simulink library "aerosimlib"  (Simulink 5.0)
values from neighbouring files (symbols this model uses):
  stdatm = [0 100 200 300 400 500 600 700 800 900 1000 1100 ... (4305 elements, 861x5)]    [stdatm.mat]
undefined symbols (not defined in the file or in its folder): AlphaBnd, b, BetaBnd, CDda, CDde, CDdf, CDdr, CDM, CDmin, CGempty, CGgross, CL0, CLa, CLalphadot, Clbeta, Clda, CLde, CLdf, Cldr, CLM, CLmind, Clp, CLq, Clr, Cm0, Cma, Cmalphadot, Cmde, Cmdf, CmM, Cmq, Cnbeta, Cnda, Cndr, Cnp, Cnr, CP, CT, CYbeta, CYda, CYdr, CYp, CYr, Displacement, dmy, Engine, EulerIni, FuelFlow, FuelIni, J, Jempty, Jeng, Jgross, Jprop, MAC, MAP, MAPLim, MassIni, MaxPower, mempty ... (+25)
libraries: aerosimlib x350, simulink3 x41
(part 5 of 10)

== system aerosimlib/Sensors/Noise Correlation ==
  Gauss-Markov  Process : Subsystem  mask(Gauss-Markov Process){beta=, seed=, Var=, T=}
      mask prompts: beta "Time constant:"; seed "White-noise seed:"; Var "Variance:"; T "Sample time:"
      mask help: The Gauss-Markov process has an exponentially decreasing autocorrelation function.
      mask Help:
      | <P>The Gauss-Markov process has an exponentially decreasing autocorrelation function.</P>
      | <P><B>Block parameters:</B>
      | <LI>Time constant = the noise correlation time.
      | <LI>White-noise seed = the starting seed of the white-noise source.
      | <LI>Variance = the variance of the white-noise source.
      | <LI>Sample time = the sample time of the white-noise source.
      | </P>
  Random Walk : Subsystem  mask(Random Walk){seed=, Var=, T=}
      mask prompts: seed "White-noise seed:"; Var "Variance:"; T "Sample time:"
      mask help: The random walk is also known as the Wiener process or Brownian motion. Essentially, this is the integral of a random noise signal.
      mask Help:
      | <P>The random walk is also known as the Wiener process or Brownian motion. Essentially, this is the integral of a random noise signal.</P>
      | <P><B>Block parameters:</B>
      | <LI>White-noise seed = the starting seed of the white-noise source.
      | <LI>Variance = the variance of the white-noise source.
      | <LI>Sample time = the sample time of the white-noise source.
      | </P>

== system aerosimlib/Transformations/Body-Inertial DCM From Euler Angles ==
  note: Sources
  note: Assemble Body-Inertial DCM
  note: Output
  note: Attitude trigonometry
  Euler : Inport  PortDimensions=[3 1]
  -sin(theta) : Gain  Gain=-1  SaturateOnIntegerOverflow=on
  Demux : Demux  Outputs=3
  Math Function : Math  Operator=transpose
  Rbi Matrix : simulink3/Signals & Systems/Matrix Concatenation  numInports=3  catMethod=Horizontal
  Rbi Col1 : simulink3/Signals & Systems/Matrix Concatenation  numInports=3  catMethod=Vertical
  Rbi Col2 : simulink3/Signals & Systems/Matrix Concatenation  numInports=3  catMethod=Vertical
  Rbi Col3 : simulink3/Signals & Systems/Matrix Concatenation  numInports=3  catMethod=Vertical
  Sum2 : Sum  Inputs=+-  SaturateOnIntegerOverflow=on  InputSameDT=on
  Sum3 : Sum  SaturateOnIntegerOverflow=on  InputSameDT=on
  Sum4 : Sum  SaturateOnIntegerOverflow=on  InputSameDT=on
  Sum5 : Sum  Inputs=+-  SaturateOnIntegerOverflow=on  InputSameDT=on
  cos(phi) : Trigonometry  Operator=cos
  cos(phi)cos(psi) : Product  SaturateOnIntegerOverflow=on  InputSameDT=on
  cos(phi)cos(theta) : Product  SaturateOnIntegerOverflow=on  InputSameDT=on
  cos(phi)sin(psi) : Product  SaturateOnIntegerOverflow=on  InputSameDT=on
  cos(phi)sin(theta)cos(psi) : Product  Inputs=3  SaturateOnIntegerOverflow=on  InputSameDT=on
  cos(phi)sin(theta)sin(psi) : Product  Inputs=3  SaturateOnIntegerOverflow=on  InputSameDT=on
  cos(psi) : Trigonometry  Operator=cos
  cos(theta) : Trigonometry  Operator=cos
  cos(theta)cos(psi) : Product  SaturateOnIntegerOverflow=on  InputSameDT=on
  cos(theta)sin(psi) : Product  SaturateOnIntegerOverflow=on  InputSameDT=on
  sin(phi) : Trigonometry
  sin(phi)cos(psi) : Product  SaturateOnIntegerOverflow=on  InputSameDT=on
  sin(phi)cos(theta) : Product  SaturateOnIntegerOverflow=on  InputSameDT=on
  sin(phi)sin(psi) : Product  SaturateOnIntegerOverflow=on  InputSameDT=on
  sin(phi)sin(theta)cos(psi) : Product  Inputs=3  SaturateOnIntegerOverflow=on  InputSameDT=on
  sin(phi)sin(theta)sin(psi) : Product  Inputs=3  SaturateOnIntegerOverflow=on  InputSameDT=on
  sin(psi) : Trigonometry
  sin(theta) : Trigonometry
  DCM : Outport
  wires:
  Euler/1 -> Demux/1
  Rbi Col1/1 -> Rbi Matrix/1
  Rbi Col2/1 -> Rbi Matrix/2
  Rbi Col3/1 -> Rbi Matrix/3
  Rbi Matrix/1 -> Math Function/1
  Demux/1 -> sin(phi)/1, cos(phi)/1
  Demux/2 -> cos(theta)/1, sin(theta)/1
  Demux/3 -> cos(psi)/1, sin(psi)/1
  sin(phi)/1 -> sin(phi)sin(psi)/1, sin(phi)cos(psi)/1, sin(phi)sin(theta)sin(psi)/1, sin(phi)cos(theta)/1, sin(phi)sin(theta)cos(psi)/1
  cos(phi)/1 -> cos(phi)cos(theta)/1, cos(phi)sin(theta)sin(psi)/1, cos(phi)sin(theta)cos(psi)/1, cos(phi)cos(psi)/1, cos(phi)sin(psi)/1
  sin(theta)/1 -> cos(phi)sin(theta)cos(psi)/2, cos(phi)sin(theta)sin(psi)/2, sin(phi)sin(theta)sin(psi)/2, sin(phi)sin(theta)cos(psi)/2, -sin(theta)/1
  cos(theta)/1 -> cos(phi)cos(theta)/2, sin(phi)cos(theta)/2, cos(theta)sin(psi)/1, cos(theta)cos(psi)/1
  sin(psi)/1 -> sin(phi)sin(psi)/2, cos(phi)sin(theta)sin(psi)/3, sin(phi)sin(theta)sin(psi)/3, cos(phi)sin(psi)/2, cos(theta)sin(psi)/2
  cos(psi)/1 -> sin(phi)cos(psi)/2, cos(phi)sin(theta)cos(psi)/3, cos(phi)cos(psi)/2, sin(phi)sin(theta)cos(psi)/3, cos(theta)cos(psi)/2
  cos(phi)sin(psi)/1 -> Sum2/2
  cos(phi)cos(psi)/1 -> Sum3/2
  sin(phi)sin(theta)cos(psi)/1 -> Sum2/1
  cos(phi)sin(theta)cos(psi)/1 -> Sum4/1
  sin(phi)sin(psi)/1 -> Sum4/2
  cos(phi)sin(theta)sin(psi)/1 -> Sum5/1
  sin(phi)cos(psi)/1 -> Sum5/2
  cos(theta)cos(psi)/1 -> Rbi Col1/1
  cos(theta)sin(psi)/1 -> Rbi Col1/2
  -sin(theta)/1 -> Rbi Col1/3
  Sum2/1 -> Rbi Col2/1
  Sum3/1 -> Rbi Col2/2
  sin(phi)cos(theta)/1 -> Rbi Col2/3
  Sum4/1 -> Rbi Col3/1
  Sum5/1 -> Rbi Col3/2
  cos(phi)cos(theta)/1 -> Rbi Col3/3
  Math Function/1 -> DCM/1
  sin(phi)sin(theta)sin(psi)/1 -> Sum3/1

== system aerosimlib/Transformations/Body-Inertial DCM From Quaternions ==
  note: Output
  note: Quaternion products
  note: Assemble Body-Inertial DCM
  note: Sources
  Quaternions : Inport  PortDimensions=[4 1]
  Demux : Demux
  Demux1 : Demux
  Gain{,1..5} (6 alike) : Gain  Gain=2  SaturateOnIntegerOverflow=on
  Get DCM : Math  Operator=transpose
  Math Function : Math  Operator=square
  Rbi Matrix : simulink3/Signals & Systems/Matrix Concatenation  numInports=3  catMethod=Horizontal
  Rbi Col1 : simulink3/Signals & Systems/Matrix Concatenation  numInports=3  catMethod=Vertical
  Rbi Col2 : simulink3/Signals & Systems/Matrix Concatenation  numInports=3  catMethod=Vertical
  Rbi Col3 : simulink3/Signals & Systems/Matrix Concatenation  numInports=3  catMethod=Vertical
  Sum : Sum  Inputs=++--  SaturateOnIntegerOverflow=on  InputSameDT=on
  Sum1 : Sum  SaturateOnIntegerOverflow=on  InputSameDT=on
  Sum2 : Sum  Inputs=+-  SaturateOnIntegerOverflow=on  InputSameDT=on
  Sum3 : Sum  Inputs=+-  SaturateOnIntegerOverflow=on  InputSameDT=on
  Sum4 : Sum  Inputs=+-+-  SaturateOnIntegerOverflow=on  InputSameDT=on
  Sum5 : Sum  SaturateOnIntegerOverflow=on  InputSameDT=on
  Sum6 : Sum  SaturateOnIntegerOverflow=on  InputSameDT=on
  Sum7 : Sum  Inputs=+-  SaturateOnIntegerOverflow=on  InputSameDT=on
  Sum8 : Sum  Inputs=+--+  SaturateOnIntegerOverflow=on  InputSameDT=on
  exe0 : Product  SaturateOnIntegerOverflow=on  InputSameDT=on
  exey : Product  SaturateOnIntegerOverflow=on  InputSameDT=on
  exez : Product  SaturateOnIntegerOverflow=on  InputSameDT=on
  eye0 : Product  SaturateOnIntegerOverflow=on  InputSameDT=on
  eyez : Product  SaturateOnIntegerOverflow=on  InputSameDT=on
  eze0 : Product  SaturateOnIntegerOverflow=on  InputSameDT=on
  DCM : Outport
  wires:
  Get DCM/1 -> DCM/1
  Rbi Matrix/1 -> Get DCM/1
  Sum8/1 -> Rbi Col3/3
  Gain5/1 -> Rbi Col3/2
  Gain4/1 -> Rbi Col3/1
  Rbi Col3/1 -> Rbi Matrix/3
  Sum7/1 -> Gain5/1
  Sum6/1 -> Gain4/1
  Rbi Col2/1 -> Rbi Matrix/2
  Gain3/1 -> Rbi Col2/3
  Sum4/1 -> Rbi Col2/2
  Gain2/1 -> Rbi Col2/1
  Sum5/1 -> Gain3/1
  Sum3/1 -> Gain2/1
  Rbi Col1/1 -> Rbi Matrix/1
  Gain1/1 -> Rbi Col1/3
  Gain/1 -> Rbi Col1/2
  Sum/1 -> Rbi Col1/1
  Sum2/1 -> Gain1/1
  Sum1/1 -> Gain/1
  exe0/1 -> Sum5/2, Sum7/2
  eyez/1 -> Sum5/1, Sum7/1
  eye0/1 -> Sum2/2, Sum6/2
  exez/1 -> Sum2/1, Sum6/1
  eze0/1 -> Sum1/2, Sum3/2
  exey/1 -> Sum1/1, Sum3/1
  Math Function/1 -> Demux1/1
  Demux/4 -> eze0/1, exez/2, eyez/2
  Demux/3 -> exey/2, eye0/1, eyez/1
  Demux/2 -> exey/1, exez/1, exe0/1
  Demux/1 -> eze0/2, eye0/2, exe0/2
  Quaternions/1 -> Math Function/1, Demux/1
  Demux1/1 -> Sum/1, Sum4/1, Sum8/1
  Demux1/2 -> Sum/2, Sum4/2, Sum8/2
  Demux1/3 -> Sum/3, Sum4/3, Sum8/3
  Demux1/4 -> Sum/4, Sum4/4, Sum8/4

== system aerosimlib/Transformations/Body-Wind DCM ==
  note: Output
  note: Assemble Body-Wind DCM
  note: Trigonometric functions
  note: Sources
  WindAxesVel : Inport  PortDimensions=[3 1]
  ChSign : Gain  Gain=-1  SaturateOnIntegerOverflow=on
  ChSign1 : Gain  Gain=-1  SaturateOnIntegerOverflow=on
  ChSign2 : Gain  Gain=-1  SaturateOnIntegerOverflow=on
  Demux : Demux  Outputs=3
  Product{,1..3} (4 alike) : Product  SaturateOnIntegerOverflow=on  InputSameDT=on
  S Matrix : simulink3/Signals & Systems/Matrix Concatenation  numInports=3  catMethod=Horizontal
  S Col1 : simulink3/Signals & Systems/Matrix Concatenation  numInports=3  catMethod=Vertical
  S Col2 : simulink3/Signals & Systems/Matrix Concatenation  numInports=3  catMethod=Vertical
  S Col3 : simulink3/Signals & Systems/Matrix Concatenation  numInports=3  catMethod=Vertical
  Terminator : Terminator
  Trigonometric Function : Trigonometry
  Trigonometric Function1 : Trigonometry  Operator=cos
  Trigonometric Function2 : Trigonometry
  Trigonometric Function3 : Trigonometry  Operator=cos
  Zero : Constant  Value=0
  DCM : Outport
  wires:
  S Matrix/1 -> DCM/1
  S Col3/1 -> S Matrix/3
  S Col2/1 -> S Matrix/2
  S Col1/1 -> S Matrix/1
  ChSign2/1 -> S Col3/2
  Product2/1 -> S Col3/1
  Product3/1 -> ChSign2/1
  Zero/1 -> S Col2/3
  ChSign1/1 -> S Col1/3
  ChSign/1 -> S Col1/2
  Product/1 -> S Col1/1
  Product1/1 -> ChSign/1
  Trigonometric Function3/1 -> Product/2, S Col2/2, Product2/2
  Trigonometric Function2/1 -> Product1/2, S Col2/1, Product3/2
  Trigonometric Function1/1 -> Product/1, Product1/1, S Col3/3
  Trigonometric Function/1 -> ChSign1/1, Product2/1, Product3/1
  Demux/1 -> Terminator/1
  WindAxesVel/1 -> Demux/1
  Demux/2 -> Trigonometric Function3/1, Trigonometric Function2/1
  Demux/3 -> Trigonometric Function/1, Trigonometric Function1/1

== system aerosimlib/Transformations/Body2LTP ==
  VecB : Inport
  Euler : Inport  Port=2
  Fcn : Fcn  Expr=cos(u(5))*u(1) + sin(u(4))*sin(u(5))*u(2) + cos(u(4))*sin(u(5))*u(3)
  Fcn1 : Fcn  Expr=cos(u(4))*u(2) - sin(u(4))*u(3)
  Fcn2 : Fcn  Expr=-sin(u(5))*u(1) + sin(u(4))*cos(u(5))*u(2) + cos(u(4))*cos(u(5))*u(3)
  Mux : Mux  Inputs=2
  Mux1 : Mux  Inputs=3
  VecLTP : Outport
  wires:
  Mux1/1 -> VecLTP/1
  Fcn2/1 -> Mux1/3
  Fcn1/1 -> Mux1/2
  Fcn/1 -> Mux1/1
  Mux/1 -> Fcn1/1, Fcn2/1, Fcn/1
  Euler/1 -> Mux/2
  VecB/1 -> Mux/1

== system aerosimlib/Transformations/ECEF Position ==
  note: Trigonometric functions
  note: Sources
  note: Output
  LLA : Inport  PortDimensions=[3 1]
  Demux : Demux  Outputs=3
  Equatorial Radius : Constant  Value=6378137
  First Eccentricity : Constant  Value=0.0818191908426
  Mux : Mux  Inputs=3
  One : Constant
  Product : Product  Inputs=3  SaturateOnIntegerOverflow=on  InputSameDT=on
  Product1 : Product  Inputs=3  SaturateOnIntegerOverflow=on  InputSameDT=on
  Product3 : Product  SaturateOnIntegerOverflow=on  InputSameDT=on
  Product4 : Product  SaturateOnIntegerOverflow=on  InputSameDT=on
  Product5 : Product  Inputs=*/  SaturateOnIntegerOverflow=on  InputSameDT=on
  Product6 : Product  SaturateOnIntegerOverflow=on  InputSameDT=on
  Sum : Sum  Inputs=|++  SaturateOnIntegerOverflow=on  InputSameDT=on
  Sum1 : Sum  Inputs=++|  SaturateOnIntegerOverflow=on  InputSameDT=on
  Sum2 : Sum  Inputs=|+-  SaturateOnIntegerOverflow=on  InputSameDT=on
  Sum3 : Sum  Inputs=|+-  SaturateOnIntegerOverflow=on  InputSameDT=on
  Trigonometric Function : Trigonometry
  Trigonometric Function1 : Trigonometry  Operator=cos
  Trigonometric Function2 : Trigonometry
  Trigonometric Function3 : Trigonometry  Operator=cos
  eps^2 : Math  Operator=square
  sin(phi)^2 : Math  Operator=square
  sqrt : Math  Operator=sqrt
  ECEF : Outport
  wires:
  Mux/1 -> ECEF/1
  Product1/1 -> Mux/2
  Product/1 -> Mux/1
  Trigonometric Function3/1 -> Product/3
  Trigonometric Function2/1 -> Product1/3
  Trigonometric Function1/1 -> Product/2, Product1/2
  LLA/1 -> Demux/1
  Demux/1 -> Trigonometric Function1/1, Trigonometric Function/1
  Demux/2 -> Trigonometric Function2/1, Trigonometric Function3/1
  Product5/1 -> Product4/1, Sum1/2
  sqrt/1 -> Product5/2
  Equatorial Radius/1 -> Product5/1
  Sum3/1 -> sqrt/1
  Product6/1 -> Sum3/2
  sin(phi)^2/1 -> Product6/1
  Product4/1 -> Sum/2
  First Eccentricity/1 -> eps^2/1
  One/1 -> Sum3/1, Sum2/1
  eps^2/1 -> Product6/2, Sum2/2
  Sum2/1 -> Product4/2
  Sum/1 -> Product3/1
  Product3/1 -> Mux/3
  Demux/3 -> Sum1/1, Sum/1
  Sum1/1 -> Product/1, Product1/1
  Trigonometric Function/1 -> sin(phi)^2/1, Product3/2

== system aerosimlib/Transformations/Euler Angles From Quaternions ==
  note: Compute Euler angles
  note: Sources
  note: Quaternion products
  Quaternions : Inport  PortDimensions=[4 1]
  2pi Bound : aerosimlib/Math/2pi Bound
  Demux : Demux
  Demux1 : Demux
  Gain6 : Gain  Gain=2  SaturateOnIntegerOverflow=on
  Gain7 : Gain  Gain=2  SaturateOnIntegerOverflow=on
  Gain8 : Gain  Gain=2  SaturateOnIntegerOverflow=on
  Math Function : Math  Operator=square
  Mux : Mux  Inputs=3
  Sum10 : Sum  Inputs=+--+  SaturateOnIntegerOverflow=on  InputSameDT=on
  Sum11 : Sum  Inputs=-+  SaturateOnIntegerOverflow=on  InputSameDT=on
  Sum12 : Sum  SaturateOnIntegerOverflow=on  InputSameDT=on
  Sum13 : Sum  Inputs=++--  SaturateOnIntegerOverflow=on  InputSameDT=on
  Sum9 : Sum  SaturateOnIntegerOverflow=on  InputSameDT=on
  Trigonometric Function : Trigonometry  Operator=atan2
  Trigonometric Function1 : Trigonometry  Operator=asin
  Trigonometric Function2 : Trigonometry  Operator=atan2
  exe0 : Product  SaturateOnIntegerOverflow=on  InputSameDT=on
  exey : Product  SaturateOnIntegerOverflow=on  InputSameDT=on
  exez : Product  SaturateOnIntegerOverflow=on  InputSameDT=on
  eye0 : Product  SaturateOnIntegerOverflow=on  InputSameDT=on
  eyez : Product  SaturateOnIntegerOverflow=on  InputSameDT=on
  eze0 : Product  SaturateOnIntegerOverflow=on  InputSameDT=on
  pi Bound : aerosimlib/Math/pi Bound
  pi Bound1 : aerosimlib/Math/pi Bound
  Euler : Outport
  wires:
  Sum9/1 -> Gain6/1
  Gain6/1 -> Trigonometric Function/1
  Sum10/1 -> Trigonometric Function/2
  Sum11/1 -> Gain7/1
  Gain7/1 -> Trigonometric Function1/1
  Sum12/1 -> Gain8/1
  Gain8/1 -> Trigonometric Function2/1
  Sum13/1 -> Trigonometric Function2/2
  Trigonometric Function1/1 -> pi Bound1/1
  Trigonometric Function/1 -> pi Bound/1
  Trigonometric Function2/1 -> 2pi Bound/1
  Quaternions/1 -> Math Function/1, Demux/1
  Demux/1 -> eze0/2, eye0/2, exe0/2
  Demux/2 -> exey/1, exez/1, exe0/1
  Demux/3 -> exey/2, eye0/1, eyez/1
  Demux/4 -> eze0/1, exez/2, eyez/2
  Demux1/1 -> Sum10/1, Sum13/1
  Demux1/2 -> Sum10/2, Sum13/2
  Demux1/3 -> Sum10/3, Sum13/3
  Demux1/4 -> Sum10/4, Sum13/4
  Math Function/1 -> Demux1/1
  exey/1 -> Sum12/1
  eze0/1 -> Sum12/2
  exez/1 -> Sum11/1
  eye0/1 -> Sum11/2
  eyez/1 -> Sum9/1
  exe0/1 -> Sum9/2
  Mux/1 -> Euler/1
  pi Bound/1 -> Mux/1
  pi Bound1/1 -> Mux/2
  2pi Bound/1 -> Mux/3

== system aerosimlib/Transformations/Euler Angles  From DCM ==
  DCM : Inport  PortDimensions=[3 3]
  C12 : Selector  InputType=Matrix  Elements=[1 3]  Columns=2  InputPortWidth=3
  C13 : Selector  InputType=Matrix  Elements=[1 3]  Columns=3  InputPortWidth=3
  C23 : Selector  InputType=Matrix  Elements=[1 3]  Rows=2  Columns=3  InputPortWidth=3
  ChSign : Gain  Gain=-1  SaturateOnIntegerOverflow=on
  Mux3 : Mux  Inputs=3
  Product2 : Product  Inputs=*/  SaturateOnIntegerOverflow=on  InputSameDT=on
  Product3 : Product  Inputs=*/  SaturateOnIntegerOverflow=on  InputSameDT=on
  Trigonometric Function : Trigonometry  Operator=asin
  Trigonometric Function1 : Trigonometry  Operator=cos
  Trigonometric Function2 : Trigonometry  Operator=asin
  Trigonometric Function3 : Trigonometry  Operator=asin
  Euler : Outport
  wires:
  DCM/1 -> C12/1, C23/1, C13/1
  Mux3/1 -> Euler/1
  Trigonometric Function3/1 -> Mux3/1
  Trigonometric Function2/1 -> Mux3/3
  Product2/1 -> Trigonometric Function2/1
  Product3/1 -> Trigonometric Function3/1
  C23/1 -> Product3/1
  Trigonometric Function1/1 -> Product3/2, Product2/2
  C12/1 -> Product2/1
  Trigonometric Function/1 -> Mux3/2, Trigonometric Function1/1
  ChSign/1 -> Trigonometric Function/1
  C13/1 -> ChSign/1

== system aerosimlib/Transformations/LTP2Body ==
  VecLTP : Inport
  Euler : Inport  Port=2
  Fcn : Fcn  Expr=cos(u(5))*u(1) - sin(u(5))*u(3)
  Fcn1 : Fcn  Expr=sin(u(4))*sin(u(5))*u(1) + cos(u(4))*u(2) + sin(u(4))*cos(u(5))*u(3)
  Fcn2 : Fcn  Expr=cos(u(4))*sin(u(5))*u(1) - sin(u(4))*u(2) + cos(u(4))*cos(u(5))*u(3)
  Mux : Mux  Inputs=2
  Mux1 : Mux  Inputs=3
  VecB : Outport
  wires:
  Mux1/1 -> VecB/1
  Fcn2/1 -> Mux1/3
  Fcn1/1 -> Mux1/2
  Fcn/1 -> Mux1/1
  Mux/1 -> Fcn1/1, Fcn2/1, Fcn/1
  Euler/1 -> Mux/2
  VecLTP/1 -> Mux/1

== system aerosimlib/Transformations/Quaternions From Euler Angles ==
  note: Sources
  note: Attitude trigonometry
  note: Compute quaternions
  note: Outputs
  Euler : Inport  PortDimensions=[3 1]
  1/2 : Gain  Gain=1/2  SaturateOnIntegerOverflow=on
  CCC : Product  Inputs=3  SaturateOnIntegerOverflow=on  InputSameDT=on
  CCS : Product  Inputs=3  SaturateOnIntegerOverflow=on  InputSameDT=on
  CSC : Product  Inputs=3  SaturateOnIntegerOverflow=on  InputSameDT=on
  CSS : Product  Inputs=3  SaturateOnIntegerOverflow=on  InputSameDT=on
  Demux : Demux  Outputs=3
  Mux : Mux
  SCC : Product  Inputs=3  SaturateOnIntegerOverflow=on  InputSameDT=on
  SCS : Product  Inputs=3  SaturateOnIntegerOverflow=on  InputSameDT=on
  SSC : Product  Inputs=3  SaturateOnIntegerOverflow=on  InputSameDT=on
  SSS : Product  Inputs=3  SaturateOnIntegerOverflow=on  InputSameDT=on
  Sum1 : Sum  SaturateOnIntegerOverflow=on  InputSameDT=on
  Sum2 : Sum  Inputs=+-  SaturateOnIntegerOverflow=on  InputSameDT=on
  Sum3 : Sum  Inputs=+-  SaturateOnIntegerOverflow=on  InputSameDT=on
  Sum9 : Sum  SaturateOnIntegerOverflow=on  InputSameDT=on
  cos(phi/2) : Trigonometry  Operator=cos
  cos(psi/2) : Trigonometry  Operator=cos
  cos(theta/2) : Trigonometry  Operator=cos
  sin(phi/2) : Trigonometry
  sin(psi/2) : Trigonometry
  sin(theta/2) : Trigonometry
  Quaternions : Outport
  wires:
  Mux/1 -> Quaternions/1
  Euler/1 -> 1/2/1
  1/2/1 -> Demux/1
  Demux/1 -> sin(phi/2)/1, cos(phi/2)/1
  Demux/2 -> cos(theta/2)/1, sin(theta/2)/1
  Demux/3 -> cos(psi/2)/1, sin(psi/2)/1
  cos(psi/2)/1 -> CCC/3, SCC/3, SSC/3, CSC/3
  sin(psi/2)/1 -> SSS/3, CSS/3, CCS/3, SCS/3
  cos(theta/2)/1 -> SCC/2, CCS/2, SCS/2, CCC/2
  sin(theta/2)/1 -> SSS/2, CSS/2, SSC/2, CSC/2
  cos(phi/2)/1 -> CSS/1, CCS/1, CSC/1, CCC/1
  sin(phi/2)/1 -> SCC/1, SSC/1, SCS/1, SSS/1
  CCC/1 -> Sum9/1
  SSS/1 -> Sum9/2
  CSC/1 -> Sum1/1
  SCS/1 -> Sum1/2
  SCC/1 -> Sum2/1
  CSS/1 -> Sum2/2
  CCS/1 -> Sum3/1
  SSC/1 -> Sum3/2
  Sum9/1 -> Mux/1
  Sum2/1 -> Mux/2
  Sum1/1 -> Mux/3
  Sum3/1 -> Mux/4

== system aerosimlib/Unit Conversion/Angular position ==
  deg 2 rad : Subsystem
      mask Type: Deg to rad
      mask Description: Convert degrees to radians.
      mask Help:
      | Degrees to radians conversion.
      | <P><B>Input:</B> angle in degrees;</P>
      | <P><B>Output:</B> angle in radians.</P>
      mask Display: disp('DEG RAD');
  rad 2 deg : Subsystem
      mask Type: Radians to degrees
      mask Description: Convert radians to degrees.
      mask Help:
      | Radians to degrees conversion.
      | <P><B>Input:</B> angle in radians;</P>
      | <P><B>Output:</B> angle in degrees.</P>
      mask Display: disp('RAD DEG');

== system aerosimlib/Unit Conversion/Angular velocity ==
  RPM 2 rad/s : Subsystem
      mask Type: RPM to rad/s
      mask Description: Convert rotations-per-minute to radians-per-second.
      mask Help:
      | Rotations per minute to radians per second conversion.
      | <P><B>Input:</B> angular speed in rotations per minute;</P>
      | <P><B>Output:</B> angular speed in radians per second.</P>
  rad/s 2 RPM : Subsystem
      mask Type: rad/s to RPM
      mask Description: Convert radians-per-second to rotations-per-minute.
      mask Help:
      | Radians per second to rotations per minute conversion.
      | <P><B>Input:</B> angular speed in radians per second;</P>
      | <P><B>Output:</B> angular speed in rotations per minute.</P>

== system aerosimlib/Unit Conversion/Distance ==
  ft 2 m : Subsystem
      mask Type: Feet to meters
      mask Description: Convert feet to meters.
      mask Help:
      | Feet to meters conversion.
      | <P><B>Input:</B> distance in feet;</P>
      | <P><B>Output:</B> distance in meters.</P>
      mask Display: disp('FT       M');
  m 2 ft : Subsystem
      mask Type: Meters to feet
      mask Description: Convert meters to feet.
      mask Help:
      | Meters to feet conversion.
      | <P><B>Input:</B> distance in meters;</P>
      | <P><B>Output:</B> distance in feet.</P>
      mask Display: disp('M       FT');
  m 2 nm : Subsystem
      mask Type: Meters to nautical miles
      mask Description: Convert meters to nautical miles.
      mask Help:
      | Meters to nautical miles conversion.
      | <P><B>Input:</B> distance in meters;</P>
      | <P><B>Output:</B> distance in nautical miles.</P>
      mask Display: disp('M       NM');
  nm 2 m : Subsystem
      mask Type: Nautical miles to meters
      mask Description: Convert nautical miles to meters.
      mask Help:
      | Nautical miles to meters conversion.
      | <P><B>Input:</B> distance in nautical miles;</P>
      | <P><B>Output:</B> distance in meters.</P>
      mask Display: disp('NM       M');

== system aerosimlib/Unit Conversion/Force ==
  N 2 lbf : Subsystem
      mask Type: Newtons to pounds
      mask Description: Convert newtons to pounds-force.
      mask Help:
      | Newton to pound conversion.
      | <P><B>Input:</B> force in newtons;</P>
      | <P><B>Output:</B> force in pounds.</P>
      mask Display: disp('N       lbf');
  lbf 2 N : Subsystem
      mask Type: Pounds to newtons
      mask Description: Convert pounds-force to newtons.
      mask Help:
      | Pound to newton conversion.
      | <P><B>Input:</B> force in pounds;</P>
      | <P><B>Output:</B> force in newtons.</P>
      mask Display: disp('lbf       N');

== system aerosimlib/Unit Conversion/Mass ==
  kg 2 lb : Subsystem
      mask Type: Kilograms to pounds
      mask Description: Convert kilograms to pounds.
      mask Help:
      | Kilograms to pounds conversion.
      | <P><B>Input:</B> mass in kilograms;</P>
      | <P><B>Output:</B> weight in pounds (at sea-level).</P>
      mask Display: disp(['__________';'          ';'KG        ';'        LB';'g         ';'----------']);
  kg 2 slug : Subsystem
      mask Type: Kilograms to slugs
      mask Description: Convert kilograms to slugs.
      mask Help:
      | Kilogram to slug conversion.
      | <P><B>Input:</B> mass in kilograms;</P>
      | <P><B>Output:</B> mass in slugs.</P>
      mask Display: disp('kg     slug');
  lb 2 kg : Subsystem
      mask Type: Pounds to kilograms
      mask Description: Convert pounds to kilograms.
      mask Help:
      | Pounds to kilograms conversion.
      | <P><B>Input:</B> weight in pounds (at sea-level);</P>
      | <P><B>Output:</B> mass in kilograms.</P>
      mask Display: disp(['__________';'          ';'LB        ';'        KG';'g         ';'----------']);
  slug 2 kg : Subsystem
      mask Type: Slugs to kilograms
      mask Description: Convert slugs to kilograms.
      mask Help:
      | Slug to kilogram conversion.
      | <P><B>Input:</B> mass in slugs;</P>
      | <P><B>Output:</B> mass in kilograms.</P>
      mask Display: disp('slug     kg');

== system aerosimlib/Unit Conversion/Pressure ==
  Pa2inHg : Subsystem
      mask Type: Pa to in.Hg
      mask Description: Convert pressure from Pascals to inches Hg.
      mask Help:
      | Convert pressure from Pascals to inches Hg.
      | <P><B>Input:</B> pressure in Pascals;</P>
      | <P><B>Output:</B> pressure in inches Hg.</P>
  inHg2Pa : Subsystem
      mask Type: in. Hg to Pa
      mask Description: Convert pressure from inches Hg to Pascals.
      mask Help:
      | Convert pressure from inches Hg to Pascals.
      | <P><B>Input:</B> pressure in inches Hg;</P>
      | <P><B>Output:</B> pressure in Pascals.</P>

== system aerosimlib/Unit Conversion/Temperature ==
  F2K : Subsystem
      mask Type: Degrees F to degrees K
      mask Description: Convert temperature from degrees Fahrenheit to degrees Kelvin.
      mask Help:
      | Convert temperature from degrees Fahrenheit to degrees Kelvin.
      | <P><B>Input:</B> temperature in degrees Fahrenheit;</P>
      | <P><B>Output:</B> temperature in degrees Kelvin.</P>
  K2F : Subsystem
      mask Type: Degrees K to degrees F
      mask Description: Convert temperature from degrees Kelvin to degrees Fahrenheit.
      mask Help:
      | Convert temperature from degrees Kelvin to degrees Fahrenheit.
      | <P><B>Input:</B> temperature in degrees Kelvin;</P>
      | <P><B>Output:</B> temperature in degrees Fahrenheit.</P>

== system aerosimlib/Unit Conversion/Velocity ==
  km/h 2 m/s : Subsystem
      mask Type: Kilometers per hour to meters per second
      mask Description: Convert kilometers per hour to meters per second.
      mask Help:
      | Kilometers per hour to meters per second conversion.
      | <P><B>Input:</B> speed in kilometers per hour;</P>
      | <P><B>Output:</B> speed in meters per second.</P>
      mask Display: disp('KM/H M/S');
  kts 2 m/s : Subsystem
      mask Type: Knots to meters per second
      mask Description: Convert knots to meters per second.
      mask Help:
      | Knots to meters per second conversion.
      | <P><B>Input:</B> speed in knots;</P>
      | <P><B>Output:</B> speed in meters per second.</P>
      mask Display: disp('KTS  M/S');
  m/s 2 km/h : Subsystem
      mask Type: Meters per second to kilometers per hour
      mask Description: Convert meters per second to kilometers per hour.
      mask Help:
      | Meters per second to kilometers per hour conversion.
      | <P><B>Input:</B> speed in meters per second;</P>
      | <P><B>Output:</B> speed in kilometers per hour.</P>
      mask Display: disp('M/S KM/H');
  m/s 2 kts : Subsystem
      mask Type: Meters per second to knots
      mask Description: Convert meters per second to knots.
      mask Help:
      | Meters per second to knots conversion.
      | <P><B>Input:</B> speed in meters per second;</P>
      | <P><B>Output:</B> speed in knots.</P>
      mask Display: disp('M/S  KTS');
  m/s 2 mph : Subsystem
      mask Type: Meters per second to miles per hour
      mask Description: Convert meters per second to miles per hour.
      mask Help:
      | Meters per second to miles per hour conversion.
      | <P><B>Input:</B> speed in meters per second;</P>
      | <P><B>Output:</B> speed in miles per hour.</P>
      mask Display: disp('M/S MPH');
  mph 2 m/s : Subsystem
      mask Type: Miles per hour to meters per second
      mask Description: Convert miles per hour to meters per second.
      mask Help:
      | Miles per hour to meters per second conversion.
      | <P><B>Input:</B> speed in miles per hour;</P>
      | <P><B>Output:</B> speed in meters per second.</P>
      mask Display: disp('MPH M/S');

== system aerosimlib/Unit Conversion/Volume ==
  gal 2 l : Subsystem
      mask Type: Gallons to liters
      mask Description: Convert gallons to liters.
      mask Help:
      | Gallon to liter conversion.
      | <P><B>Input:</B> volume in gallons;</P>
      | <P><B>Output:</B> volume in liters.</P>
      mask Display: disp('gal       l');
  l 2 gal : Subsystem
      mask Type: Liters to gallons
      mask Description: Convert liters to gallons.
      mask Help:
      | Liter to gallon conversion.
      | <P><B>Input:</B> volume in liters;</P>
      | <P><B>Output:</B> volume in gallons.</P>
      mask Display: disp('l       gal');

== system aerosimlib/Atmosphere/Turbulence/Lateral  Turbulence Filter ==
  note: Outputs
  note: Filter dynamics
  note: Build state space model
  note: Matrix elements
  note: Sources
  Airspeed : Inport  PortDimensions=1
  RefLength : Inport  Port=2  PortDimensions=1
  Intensity : Inport  Port=3  PortDimensions=1
  A : simulink3/Signals & Systems/Matrix Concatenation  numInports=2  catMethod=Vertical
  A row 1 : simulink3/Signals & Systems/Matrix Concatenation  numInports=2  catMethod=Horizontal
  A row 2 : simulink3/Signals & Systems/Matrix Concatenation  numInports=2  catMethod=Horizontal
  Ax : Product  Multiplication=Matrix(*)  SaturateOnIntegerOverflow=on  InputSameDT=on
  B : simulink3/Signals & Systems/Matrix Concatenation  numInports=2  catMethod=Vertical
  Bu : Product  Multiplication=Matrix(*)  SaturateOnIntegerOverflow=on  InputSameDT=on
  C : simulink3/Signals & Systems/Matrix Concatenation  numInports=2  catMethod=Horizontal
  Constant : Constant  Value=0
  Constant1 : Constant
  Cx : Product  Multiplication=Matrix(*)  SaturateOnIntegerOverflow=on  InputSameDT=on
  Derivative : Derivative
  Gain : Gain  Gain=2  SaturateOnIntegerOverflow=on
  Gain1 : Gain  Gain=-28.84  SaturateOnIntegerOverflow=on
  Gain2 : Gain  Gain=1.776  SaturateOnIntegerOverflow=on
  Gain3 : Gain  Gain=-26.51  SaturateOnIntegerOverflow=on
  Gain4 : Gain  Gain=26.51  SaturateOnIntegerOverflow=on
  Integrator : Integrator  InitialCondition=zeros(2,1)
  Math Function : Math  Operator=square
  Math Function1 : Math  Operator=sqrt
  Product : Product  Inputs=*/  SaturateOnIntegerOverflow=on  InputSameDT=on
  Product1 : Product  Inputs=*/  SaturateOnIntegerOverflow=on  InputSameDT=on
  Product2 : Product  SaturateOnIntegerOverflow=on  InputSameDT=on
  Sum : Sum  Inputs=|++  SaturateOnIntegerOverflow=on  InputSameDT=on
  White Noise : RandomNumber  Seed=[32412]  SampleTime=tsamp
  LatVel : Outport
  LatAcc : Outport  Port=2
  wires:
  Integrator/1 -> Cx/2, Ax/2
  Intensity/1 -> Product2/2
  Derivative/1 -> LatAcc/1
  Cx/1 -> Derivative/1, LatVel/1
  Bu/1 -> Sum/2
  White Noise/1 -> Bu/2
  Sum/1 -> Integrator/1
  Ax/1 -> Sum/1
  C/1 -> Cx/1
  B/1 -> Bu/1
  A/1 -> Ax/1
  A row 2/1 -> A/2
  A row 1/1 -> A/1
  Constant/1 -> B/2, A row 2/2
  Constant1/1 -> A row 2/1
  Product2/1 -> B/1
  Math Function1/1 -> Product2/1
  Gain4/1 -> C/2
  Gain3/1 -> A row 1/2
  Math Function/1 -> Gain4/1, Gain3/1
  Gain2/1 -> C/1
  Gain1/1 -> A row 1/1
  Gain/1 -> Math Function1/1
  Product/1 -> Gain2/1, Gain1/1, Math Function/1
  Product1/1 -> Gain/1
  RefLength/1 -> Product/2, Product1/1
  Airspeed/1 -> Product/1, Product1/2

== system aerosimlib/Atmosphere/Turbulence/Longitudinal  Turbulence Filter ==
  note: Sources
  note: Matrix elements
  note: Build state space model
  note: Filter dynamics
  note: Outputs
  Airspeed : Inport  PortDimensions=1
  RefLength : Inport  Port=2  PortDimensions=1
  Intensity : Inport  Port=3  PortDimensions=1
  A : simulink3/Signals & Systems/Matrix Concatenation  numInports=2  catMethod=Vertical
  A row 1 : simulink3/Signals & Systems/Matrix Concatenation  numInports=2  catMethod=Horizontal
  A row 2 : simulink3/Signals & Systems/Matrix Concatenation  numInports=2  catMethod=Horizontal
  Ax : Product  Multiplication=Matrix(*)  SaturateOnIntegerOverflow=on  InputSameDT=on
  B : simulink3/Signals & Systems/Matrix Concatenation  numInports=2  catMethod=Vertical
  Bu : Product  Multiplication=Matrix(*)  SaturateOnIntegerOverflow=on  InputSameDT=on
  C : simulink3/Signals & Systems/Matrix Concatenation  numInports=2  catMethod=Horizontal
  Constant : Constant  Value=0
  Constant1 : Constant
  Cx : Product  Multiplication=Matrix(*)  SaturateOnIntegerOverflow=on  InputSameDT=on
  Derivative : Derivative
  Gain : Gain  Gain=2  SaturateOnIntegerOverflow=on
  Gain1 : Gain  Gain=-28.84  SaturateOnIntegerOverflow=on
  Gain2 : Gain  Gain=1.776  SaturateOnIntegerOverflow=on
  Gain3 : Gain  Gain=-26.51  SaturateOnIntegerOverflow=on
  Gain4 : Gain  Gain=26.51  SaturateOnIntegerOverflow=on
  Integrator : Integrator  InitialCondition=zeros(2,1)
  Math Function : Math  Operator=square
  Math Function1 : Math  Operator=sqrt
  Product : Product  Inputs=*/  SaturateOnIntegerOverflow=on  InputSameDT=on
  Product1 : Product  Inputs=*/  SaturateOnIntegerOverflow=on  InputSameDT=on
  Product2 : Product  SaturateOnIntegerOverflow=on  InputSameDT=on
  Sum : Sum  Inputs=|++  SaturateOnIntegerOverflow=on  InputSameDT=on
  White Noise : RandomNumber  Seed=[12344]  SampleTime=tsamp
  LongVel : Outport
  LongAcc : Outport  Port=2
  wires:
  Airspeed/1 -> Product1/2, Product/1
  RefLength/1 -> Product1/1, Product/2
  Product1/1 -> Gain/1
  Product/1 -> Math Function/1, Gain1/1, Gain2/1
  Gain/1 -> Math Function1/1
  Gain1/1 -> A row 1/1
  Gain2/1 -> C/1
  Math Function/1 -> Gain3/1, Gain4/1
  Gain3/1 -> A row 1/2
  Gain4/1 -> C/2
  Math Function1/1 -> Product2/1
  Product2/1 -> B/1
  Constant1/1 -> A row 2/1
  Constant/1 -> A row 2/2, B/2
  A row 1/1 -> A/1
  A row 2/1 -> A/2
  A/1 -> Ax/1
  B/1 -> Bu/1
  C/1 -> Cx/1
  Ax/1 -> Sum/1
  Sum/1 -> Integrator/1
  White Noise/1 -> Bu/2
  Bu/1 -> Sum/2
  Cx/1 -> LongVel/1, Derivative/1
  Derivative/1 -> LongAcc/1
  Intensity/1 -> Product2/2
  Integrator/1 -> Ax/2, Cx/2

== system aerosimlib/Atmosphere/Turbulence/Turbulence Characteristics ==
  note: Sources
  note: Outputs
  AGLAlt : Inport  PortDimensions=1
  WindVel : Inport  Port=2  PortDimensions=[3 1]
  Constant : Constant  Value=0.177
  Constant1 : Constant  Value=0.4
  Constant2 : Constant  Value=1.2
  Constant3 : Constant  Value=75.6
  Constant4 : Constant  Value=10
  Constant5 : Constant  Value=1000
  Gain : Gain  Gain=0.1  SaturateOnIntegerOverflow=on
  Gain1 : Gain  Gain=0.000823  SaturateOnIntegerOverflow=on
  Math Function : Math  Operator=pow
  Math Function1 : Math  Operator=pow
  Product : Product  Inputs=*/  SaturateOnIntegerOverflow=on  InputSameDT=on
  Product1 : Product  Inputs=*/  SaturateOnIntegerOverflow=on  InputSameDT=on
  Sum : Sum  Inputs=|++  SaturateOnIntegerOverflow=on  InputSameDT=on
  Switch : Switch  Threshold=1000  SaturateOnIntegerOverflow=on  InputSameDT=on
  Switch1 : Switch  Threshold=1000  SaturateOnIntegerOverflow=on  InputSameDT=on
  Switch2 : Switch  Threshold=1000  SaturateOnIntegerOverflow=on  InputSameDT=on
  Switch3 : Switch  Threshold=10  SaturateOnIntegerOverflow=on  InputSameDT=on
  Switch4 : Switch  Threshold=10  SaturateOnIntegerOverflow=on  InputSameDT=on
  Switch5 : Switch  Threshold=10  SaturateOnIntegerOverflow=on  InputSameDT=on
  Vector norm : Subsystem
      mask Type: Vector norm-2
      mask Description: Compute the 2-norm (magnitude) of a vector, |v| = sqrt(v'v).
  sigmau : Outport
  sigmav : Outport  Port=2
  sigmaw : Outport  Port=3
  Lu : Outport  Port=4
  Lv : Outport  Port=5
  Lw : Outport  Port=6
  wires:
  AGLAlt/1 -> Switch/2, Switch1/2, Switch2/2, Switch3/2, Switch4/2, Switch5/2, Switch5/1, Product1/1, Gain1/1
  WindVel/1 -> Vector norm/1(Vec)
  Gain/1 -> Product/1, sigmaw/1
  Constant/1 -> Sum/1
  Gain1/1 -> Sum/2
  Sum/1 -> Math Function/1, Math Function1/1
  Constant1/1 -> Math Function/2
  Constant2/1 -> Math Function1/2
  Constant4/1 -> Switch5/3
  Constant5/1 -> Switch2/1, Switch1/1, Switch/1
  Switch3/1 -> Switch/3
  Switch4/1 -> Switch1/3
  Switch5/1 -> Switch2/3
  Switch/1 -> Lu/1
  Switch1/1 -> Lv/1
  Switch2/1 -> Lw/1
  Product1/1 -> Switch3/1, Switch4/1
  Constant3/1 -> Switch4/3, Switch3/3
  Math Function/1 -> Product/2
  Math Function1/1 -> Product1/2
  Vector norm/1(Mag) -> Gain/1
  Product/1 -> sigmau/1, sigmav/1

== system aerosimlib/Atmosphere/Turbulence/Vertical  Turbulence Filter ==
  note: Sources
  note: Matrix elements
  note: Build state space model
  note: Filter dynamics
  note: Outputs
  Airspeed : Inport  PortDimensions=1
  RefLength : Inport  Port=2  PortDimensions=1
  Intensity : Inport  Port=3  PortDimensions=1
  A : simulink3/Signals & Systems/Matrix Concatenation  numInports=2  catMethod=Vertical
  A row 1 : simulink3/Signals & Systems/Matrix Concatenation  numInports=2  catMethod=Horizontal
  A row 2 : simulink3/Signals & Systems/Matrix Concatenation  numInports=2  catMethod=Horizontal
  Ax : Product  Multiplication=Matrix(*)  SaturateOnIntegerOverflow=on  InputSameDT=on
  B : simulink3/Signals & Systems/Matrix Concatenation  numInports=2  catMethod=Vertical
  Bu : Product  Multiplication=Matrix(*)  SaturateOnIntegerOverflow=on  InputSameDT=on
  C : simulink3/Signals & Systems/Matrix Concatenation  numInports=2  catMethod=Horizontal
  Constant : Constant  Value=0
  Constant1 : Constant
  Cx : Product  Multiplication=Matrix(*)  SaturateOnIntegerOverflow=on  InputSameDT=on
  Derivative : Derivative
  Gain : Gain  Gain=2  SaturateOnIntegerOverflow=on
  Gain1 : Gain  Gain=-28.84  SaturateOnIntegerOverflow=on
  Gain2 : Gain  Gain=1.776  SaturateOnIntegerOverflow=on
  Gain3 : Gain  Gain=-26.51  SaturateOnIntegerOverflow=on
  Gain4 : Gain  Gain=26.51  SaturateOnIntegerOverflow=on
  Integrator : Integrator  InitialCondition=zeros(2,1)
  Math Function : Math  Operator=square
  Math Function1 : Math  Operator=sqrt
  Product : Product  Inputs=*/  SaturateOnIntegerOverflow=on  InputSameDT=on
  Product1 : Product  Inputs=*/  SaturateOnIntegerOverflow=on  InputSameDT=on
  Product2 : Product  SaturateOnIntegerOverflow=on  InputSameDT=on
  Sum : Sum  Inputs=|++  SaturateOnIntegerOverflow=on  InputSameDT=on
  White Noise : RandomNumber  Seed=[44231]  SampleTime=tsamp
  VertVel : Outport
  VertAcc : Outport  Port=2
  wires:
  Airspeed/1 -> Product1/2, Product/1
  RefLength/1 -> Product1/1, Product/2
  Product1/1 -> Gain/1
  Product/1 -> Math Function/1, Gain1/1, Gain2/1
  Gain/1 -> Math Function1/1
  Gain1/1 -> A row 1/1
  Gain2/1 -> C/1
  Math Function/1 -> Gain3/1, Gain4/1
  Gain3/1 -> A row 1/2
  Gain4/1 -> C/2
  Math Function1/1 -> Product2/1
  Product2/1 -> B/1
  Constant1/1 -> A row 2/1
  Constant/1 -> A row 2/2, B/2
  A row 1/1 -> A/1
  A row 2/1 -> A/2
  A/1 -> Ax/1
  B/1 -> Bu/1
  C/1 -> Cx/1
  Ax/1 -> Sum/1
  Sum/1 -> Integrator/1
  White Noise/1 -> Bu/2
  Bu/1 -> Sum/2
  Cx/1 -> VertVel/1, Derivative/1
  Derivative/1 -> VertAcc/1
  Intensity/1 -> Product2/2
  Integrator/1 -> Ax/2, Cx/2

== system aerosimlib/Atmosphere/Wind Shear/Zero Offset1 ==
  In : Inport
  Abs : Abs  SaturateOnIntegerOverflow=on
  Constant : Constant  Value=tol
  Non-zero Sign : Subsystem
      mask Type: Non-zero sign
      mask Description: Sign function outputs 1 for input greater than or equal to 0, and -1 otherwise.
  Product : Product  SaturateOnIntegerOverflow=on  InputSameDT=on
  Switch : Switch  Threshold=tol  SaturateOnIntegerOverflow=on  InputSameDT=on
  Out : Outport
  wires:
  In/1 -> Switch/1, Non-zero Sign/1(In), Abs/1
  Abs/1 -> Switch/2
  Non-zero Sign/1(Out) -> Product/1
  Constant/1 -> Product/2
  Product/1 -> Switch/3
  Switch/1 -> Out/1

== system aerosimlib/Atmosphere/Wind Shear/Zero Offset2 ==
  In : Inport
  Abs : Abs  SaturateOnIntegerOverflow=on
  Constant : Constant  Value=tol
  Non-zero Sign : Subsystem
      mask Type: Non-zero sign
      mask Description: Sign function outputs 1 for input greater than or equal to 0, and -1 otherwise.
  Product : Product  SaturateOnIntegerOverflow=on  InputSameDT=on
  Switch : Switch  Threshold=tol  SaturateOnIntegerOverflow=on  InputSameDT=on
  Out : Outport
  wires:
  Switch/1 -> Out/1
  Product/1 -> Switch/3
  Constant/1 -> Product/2
  Non-zero Sign/1(Out) -> Product/1
  Abs/1 -> Switch/2
  In/1 -> Abs/1, Non-zero Sign/1(In), Switch/1

== system aerosimlib/Complete Aircraft/6-DOF Aircraft Model (Body-frame EOM)/Aerodynamics ==
  note: Aerodynamic Loads
  note: Aerodynamic Coefficients
  note: Aerodynamic Parameters
  note: Outputs
  note: Inputs
  VelB : Inport  PortDimensions=[3 1]
  WindB : Inport  Port=2  PortDimensions=[3 1]
  Rates : Inport  Port=3  PortDimensions=[3 1]
  WindRates : Inport  Port=4  PortDimensions=[3 1]
  AeroCon : Inport  Port=5  PortDimensions=[4 1]
  rho : Inport  Port=6  PortDimensions=1
  a : Inport  Port=7  PortDimensions=1
  Aerodynamic Force : aerosimlib/Aerodynamics/Aerodynamic Force  S=S
  Aerodynamic Moment : aerosimlib/Aerodynamics/Aerodynamic Moment  c=MAC  b=b  S=S
  Drag Coefficient : aerosimlib/Aerodynamics/Drag Coefficient  CL0=CLmind  CD0=CDmin  CDdf=CDdf  CDde=CDde  CDda=CDda  CDdr=CDdr  CDM=CDM  e=osw  b=b  S=S
  Dynamic Pressure : aerosimlib/Aerodynamics/Dynamic Pressure
  Lift Coefficient : aerosimlib/Aerodynamics/Lift Coefficient  CL0=CL0  CLalpha=CLa  CLdf=CLdf  CLde=CLde  CLalphadot=CLalphadot  CLq=CLq  CLM=CLM  c=MAC
  Mux : Mux  Inputs=6
  Pitch Moment Coefficient : aerosimlib/Aerodynamics/Pitch Moment Coefficient  Cm0=Cm0  Cma=Cma  Cmdf=Cmdf  Cmde=Cmde  Cmalphadot=Cmalphadot  Cmq=Cmq  CmM=CmM  c=MAC
  Roll Moment Coefficient : aerosimlib/Aerodynamics/Roll Moment Coefficient  Clbeta=Clbeta  Clda=Clda  Cldr=Cldr  Clp=Clp  Clr=Clr  b=b
  Side Force Coefficient : aerosimlib/Aerodynamics/Side Force Coefficient  CYbeta=CYbeta  CYda=CYda  CYdr=CYdr  CYp=CYp  CYr=CYr  b=b
  Sum : Sum  Inputs=|+-  SaturateOnIntegerOverflow=on  InputSameDT=on
  Wind-axes Velocities : aerosimlib/Aerodynamics/Wind-axes Velocities  Vabnd=VaBnd  betabnd=BetaBnd  alphabnd=AlphaBnd
  Yaw Moment Coefficient : aerosimlib/Aerodynamics/Yaw Moment Coefficient  Cnbeta=Cnbeta  Cnda=Cnda  Cndr=Cndr  Cnp=Cnp  Cnr=Cnr  b=b
  Faero : Outport
  Maero : Outport  Port=2
  AeroCoeff : Outport  Port=3
  VelW : Outport  Port=4
  Mach : Outport  Port=5
  pdyn : Outport  Port=6
  wires:
  VelB/1 -> Wind-axes Velocities/1
  WindB/1 -> Wind-axes Velocities/2
  a/1 -> Wind-axes Velocities/3
  Wind-axes Velocities/1 -> Lift Coefficient/1, Dynamic Pressure/1, Drag Coefficient/1, Side Force Coefficient/1, Pitch Moment Coefficient/1, Roll Moment Coefficient/1, Yaw Moment Coefficient/1, Aerodynamic Force/5, VelW/1
  rho/1 -> Dynamic Pressure/2
  AeroCon/1 -> Lift Coefficient/2, Drag Coefficient/2, Side Force Coefficient/2, Pitch Moment Coefficient/2, Roll Moment Coefficient/2, Yaw Moment Coefficient/2
  Wind-axes Velocities/2 -> Lift Coefficient/3, Pitch Moment Coefficient/3
  Wind-axes Velocities/3 -> Drag Coefficient/4, Pitch Moment Coefficient/5, Lift Coefficient/5, Mach/1
  Lift Coefficient/1 -> Aerodynamic Force/3, Drag Coefficient/3, Mux/3
  Drag Coefficient/1 -> Aerodynamic Force/1, Mux/1
  Side Force Coefficient/1 -> Aerodynamic Force/2, Mux/2
  Dynamic Pressure/1 -> Aerodynamic Force/4, Aerodynamic Moment/4, pdyn/1
  Roll Moment Coefficient/1 -> Aerodynamic Moment/1, Mux/4
  Pitch Moment Coefficient/1 -> Aerodynamic Moment/2, Mux/5
  Yaw Moment Coefficient/1 -> Aerodynamic Moment/3, Mux/6
  Aerodynamic Force/1 -> Faero/1
  Aerodynamic Moment/1 -> Maero/1
  Mux/1 -> AeroCoeff/1
  Rates/1 -> Sum/1
  WindRates/1 -> Sum/2
  Sum/1 -> Lift Coefficient/4, Side Force Coefficient/3, Pitch Moment Coefficient/4, Yaw Moment Coefficient/3, Roll Moment Coefficient/3

== system aerosimlib/Complete Aircraft/6-DOF Aircraft Model (Body-frame EOM)/Atmosphere ==
  note: Inputs
  note: Outputs
  MSL : Inport  PortDimensions=1  DataType=double
  AGL : Inport  Port=2  PortDimensions=1  DataType=double
  Winds : Inport  Port=3  PortDimensions=[3 1]  DataType=double
  VelB : Inport  Port=4  PortDimensions=[3 1]  DataType=double
  VelW : Inport  Port=5  PortDimensions=[3 1]
  DCM : Inport  Port=6  PortDimensions=[3 3]  DataType=double
  Background Wind : aerosimlib/Atmosphere/Background Wind
  Standard Atmosphere : aerosimlib/Atmosphere/Standard Atmosphere
  Sum : Sum  Inputs=|++  SaturateOnIntegerOverflow=on  InputSameDT=on
  Terminator : Terminator
  Turbulence : aerosimlib/Atmosphere/Turbulence  tsamp=tsamp
  Wind Shear : aerosimlib/Atmosphere/Wind Shear
  pstatic : Outport
  OAT : Outport  Port=2
  rho : Outport  Port=3
  a : Outport  Port=4
  WindVel : Outport  Port=5
  WindRates : Outport  Port=6
  wires:
  MSL/1 -> Standard Atmosphere/1
  Winds/1 -> Background Wind/1
  DCM/1 -> Background Wind/2
  Background Wind/1 -> Turbulence/3, Sum/2
  AGL/1 -> Turbulence/2
  VelW/1 -> Turbulence/1
  Background Wind/2 -> Wind Shear/1
  Turbulence/1 -> Sum/1
  Turbulence/2 -> Wind Shear/2
  VelB/1 -> Wind Shear/3
  Wind Shear/1 -> WindRates/1
  Standard Atmosphere/1 -> pstatic/1
  Standard Atmosphere/2 -> OAT/1
  Standard Atmosphere/3 -> rho/1
  Standard Atmosphere/4 -> a/1
  Sum/1 -> WindVel/1
  Wind Shear/2 -> Terminator/1

== system aerosimlib/Complete Aircraft/6-DOF Aircraft Model (Body-frame EOM)/Earth ==
  note: Inputs
  note: Outputs
  Position : Inport  PortDimensions=[3 1]  DataType=double
  DCM : Inport  Port=2  PortDimensions=[3 3]  DataType=double
  ECEF Position : aerosimlib/Transformations/ECEF Position
  EGM-96 : aerosimlib/Earth/EGM-96
  Ground Alt : Constant  Value=GndAlt
  Ground Detection : aerosimlib/Earth/Ground Detection
  Mux3 : Mux  Inputs=2
  WGS-84 : aerosimlib/Earth/WGS-84
  WMM-2000 : aerosimlib/Earth/WMM-2000  wmmfile=wmmfile  simdate=dmy
  MSL : Outport
  AGL : Outport  Port=2
  AConGnd : Outport  Port=3
  Rearth : Outport  Port=4
  Requiv : Outport  Port=5
  Gravity : Outport  Port=6
  MagField : Outport  Port=7
  ECEF : Outport  Port=8
  wires:
  Position/1 -> WGS-84/1, EGM-96/1, WMM-2000/1, ECEF Position/1
  DCM/1 -> WMM-2000/2
  Ground Alt/1 -> Ground Detection/2
  EGM-96/1 -> Ground Detection/1, MSL/1
  WGS-84/1 -> Mux3/1
  WGS-84/2 -> Mux3/2
  Ground Detection/2 -> AGL/1
  Ground Detection/1 -> AConGnd/1
  Mux3/1 -> Rearth/1
  WGS-84/3 -> Requiv/1
  WGS-84/4 -> Gravity/1
  WMM-2000/1 -> MagField/1
  ECEF Position/1 -> ECEF/1

== system aerosimlib/Complete Aircraft/6-DOF Aircraft Model (Body-frame EOM)/Equations of Motion ==
  note: Outputs
  note: Inputs
  Accel : Inport  PortDimensions=[3 1]
  Moment : Inport  Port=2  PortDimensions=[3 1]
  Inertia : Inport  Port=3  PortDimensions=[4 1]
  Rearth : Inport  Port=4  PortDimensions=[2 1]
  Gravity : Inport  Port=5  PortDimensions=1
  AConGnd : Inport  Port=6  PortDimensions=1
  RST : Inport  Port=7  PortDimensions=1
  Body-Inertial DCM From Quaternions : aerosimlib/Transformations/Body-Inertial DCM From Quaternions
  Demux : Demux  Outputs=2
  Euler Angles From Quaternions : aerosimlib/Transformations/Euler Angles From Quaternions
  Forces : aerosimlib/Equations of Motion/Body-Frame EOM/Forces  VelocitiesIni=VelocitiesIni
  Kinematics (Quaternions) : aerosimlib/Equations of Motion/Body-Frame EOM/Kinematics (Quaternions)  QuaternionsIni=QuaternionsIni
  Moments : aerosimlib/Equations of Motion/Body-Frame EOM/Moments  RatesIni=RatesIni
  Navigation : aerosimlib/Equations of Motion/Body-Frame EOM/Navigation  PositionIni=PositionIni
  VelB : Outport
  Rates : Outport  Port=2
  Quaternions : Outport  Port=3
  Position : Outport  Port=4
  Groundspeed : Outport  Port=5
  DCM : Outport  Port=6
  Euler : Outport  Port=7
  Ang Acc : Outport  Port=8
  wires:
  Euler Angles From Quaternions/1 -> Euler/1
  Body-Inertial DCM From Quaternions/1 -> DCM/1, Forces/4, Navigation/2
  Rearth/1 -> Demux/1
  Demux/1 -> Navigation/3
  Demux/2 -> Navigation/4
  Accel/1 -> Forces/2
  Moment/1 -> Moments/2
  Inertia/1 -> Moments/1
  Gravity/1 -> Forces/3
  AConGnd/1 -> Navigation/5
  Forces/1 -> VelB/1, Navigation/1
  Kinematics (Quaternions)/1 -> Quaternions/1, Euler Angles From Quaternions/1, Body-Inertial DCM From Quaternions/1
  Moments/1 -> Forces/1, Kinematics (Quaternions)/1, Rates/1
  RST/1 -> Forces/5, Moments/3, Navigation/6, Kinematics (Quaternions)/2
  Moments/2 -> Ang Acc/1
  Navigation/1 -> Position/1
  Navigation/2 -> Groundspeed/1
